simulink model "FromGES"  (R2016b)
settings: Solver=VariableStepAuto  StartTime=0.0  StopTime=10.0  RelTol=1e-3
settings Model: DataDictionary=ModelDictionary.sldd  Creator=Nathan  LastModifiedBy=Nathan

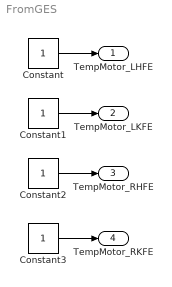
== system FromGES ==
  Constant{,1..3} (4 alike) : Constant
  TempMotor_LHFE : Outport
  TempMotor_LKFE : Outport  Port=2
  TempMotor_RHFE : Outport  Port=3
  TempMotor_RKFE : Outport  Port=4
  wires:
  Constant/1 -> TempMotor_LHFE/1
  Constant1/1 -> TempMotor_LKFE/1
  Constant2/1 -> TempMotor_RHFE/1
  Constant3/1 -> TempMotor_RKFE/1
